simulink model "model"  (R2020b)
settings: Solver=VariableStepAuto  StartTime=0.0  StopTime=10.0  RelTol=1e-3
settings Model: Creator=Arvind Hishikar  LastModifiedBy=Arvind Hishikar

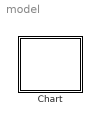
== system model ==
  Chart : Stateflow chart  TreatAsAtomicUnit=on

== stateflow chart model/Chart ==
  state Stop
    y1= RED;
    y2 = GREEN;
  state StpForTraffic
    y1 = RED;
    y2 = GREEN;
  state StopToGo
    y1= RED;
    y2 = YELOW;
  state GoToStop
    y1 = YELLOW;
    y2 = RED;
  state Go
    y1 = GREEN;
    y2 = RED;
  (default) -> Stop
  Stop -> StpForTraffic : after(20,tick)
  StpForTraffic -> StopToGo : [sensor]
  GoToStop -> Stop : after(3,tick)
  StopToGo -> Go : after(3,tick)
  Go -> GoToStop : after(10,tick)
